simulink model "hpt_v2_1to1_switchlevel"  (R2025a)
settings: Solver=ode23tb  StartTime=0.0  StopTime=0.2  RelTol=1e-3
model workspace (MAT data in the model file):
  hpt_chopper_threshold = 850
  hpt_conventional_energy_scale = 1
  hpt_conventional_energy_scale_sag = 1
  hpt_conventional_energy_scale_swell = 1
  hpt_conventional_recovery_hold_s = 0
  hpt_conventional_recovery_reg_gain = 0
  hpt_conventional_recovery_reg_max = 0
  hpt_conventional_reg_scale = 1
  hpt_conventional_reg_scale_sag = 1
  hpt_conventional_reg_scale_swell = 1
  hpt_ctrl_Ts = 2e-05
  hpt_energy_bridge_polarity = -1
  hpt_energy_control_sign = -1
  hpt_energy_i_ki = 100
  hpt_energy_i_kp = 0.5
  hpt_energy_id_max = 20
  hpt_energy_openloop_amp = 0
  hpt_energy_openloop_phase = 0
  hpt_energy_vff_gain = 1.06
  hpt_grid_f0 = 50
  hpt_inj_phase_offset = -1.05
  hpt_m_energy = 0
  hpt_m_energy_max = 0.95
  hpt_m_reg = 0.1
  hpt_m_reg_max = 0.8
  hpt_pll_ki = 2500
  hpt_pll_kp = 80
  hpt_pwm_fs = 2000
  hpt_rchop = 5.33333333333
  hpt_sac_actor_filter_tau = 0.001
  hpt_sac_actor_select_mode = 0
  hpt_sac_dynamic_reg_limit = 0.8
  hpt_sac_enable = 0
  hpt_sac_energy_enable = 0
  hpt_sac_energy_max = 0.95
  hpt_sac_fault_time_norm_s = 0.5
  hpt_sac_fixed_energy_d = 0
  hpt_sac_fixed_energy_q = 0
  hpt_sac_fixed_reg_d = 0
  hpt_sac_fixed_reg_q = 0
  hpt_sac_grid_vref_phase = 5773.5026919
  hpt_sac_gridnorm_startup_s = 0.03
  hpt_sac_guard_enable = 0
  hpt_sac_i_base_peak = 816.496580928
  hpt_sac_phase_fault_clear_s = 0
  hpt_sac_phase_fault_start_s = 0
  hpt_sac_phase_override_enable = 0
  hpt_sac_phase_recovery_end_s = 0
  hpt_sac_policy_mode = 0
  hpt_sac_recovery_time_norm_s = 0.5
  hpt_sac_reg_d_gain = 1
  hpt_sac_reg_max = 0.8
  hpt_sac_reg_polarity = 1
  hpt_sac_reg_q_gain = 1
  hpt_sac_topology_id = 1
  hpt_sac_vdc_ref = 800
  hpt_sac_vref_phase = 230
  hpt_swell_gain_scale = 1
  hpt_traj_action = [0  0  0  0; 0  0  0  0; 0  0  0  0; 0  0  0  0; 0  0  0  0; 0  0  0  0; 0  0  0  0; 0  0  0  0; 0  0  0  0; 0  0  0  0; 0  0  0  0; 0  0  0  0; 0  0  0  0; 0  0  0  0; 0  0  0  0; 0  0  0  0; 0  0  0  0; 0  0  0  0; 0  0  0  0; 0  0  0  0; 0  0  0  0; 0  0  0  0; 0  0  0  0; 0  0  0  0; 0  0  0  0; 0  0  0  0; 0  0  0  0; 0  0  0  0; 0  0  0  0; 0  0  0  0; 0  0  0  0; 0  0  0  0; 0  0  0  0; 0  0  0  0; 0  0  0  0; 0  0  0  0; 0  0  0  0; 0  0  0  0; 0  0  0  0; 0  0  0  0; 0  0  0  0; 0  0  0  0; 0  0  0  0; 0  0  0  0; 0  0  0  0; 0  0  0  0; 0  0  0  0; 0  0  0  0; 0  0  0  0; 0  0  0  0; 0  0  0  0; 0  0  0  0; 0  0  0  0; 0  0  0  0; 0  0  0  0; 0  0  0  0; 0  0  0  0; 0  0  0  0; 0  0  0  0; 0  0  0  0; 0  0  0  0; 0  0  0  0; 0  0  0  0; 0  0  0  0; 0  0  0  0; 0  0  0  0; 0  0  0  0; 0  0  0  0; 0  0  0  0; 0  0  0  0; 0  0  0  0; 0  0  0  0; 0  0  0  0; 0  0  0  0; 0  0  0  0; 0  0  0  0; 0  0  0  0; 0  0  0  0; 0  0  0  0; 0  0  0  0; 0  0  0  0; 0  0  0  0; 0  0  0  0; 0  0  0  0; 0  0  0  0; 0  0  0  0; 0  0  0  0; 0  0  0  0; 0  0  0  0; 0  0  0  0; 0  0  0  0; 0  0  0  0; 0  0  0  0; 0  0  0  0; 0  0  0  0; 0  0  0  0; 0  0  0  0; 0  0  0  0; 0  0  0  0; 0  0  0  0; 0  0  0  0; 0  0  0  0; 0  0  0  0; 0  0  0  0; 0  0  0  0; 0  0  0  0; 0  0  0  0; 0  0  0  0; 0  0  0  0; 0  0  0  0; 0  0  0  0; 0  0  0  0; 0  0  0  0; 0  0  0  0; 0  0  0  0; 0  0  0  0; 0  0  0  0; 0  0  0  0; 0  0  0  0; 0  0  0  0; 0  0  0  0; 0  0  0  0; 0  0  0  0; 0  0  0  0; 0  0  0  0; 0  0  0  0]
  hpt_traj_t = [0; 0.002; 0.004; 0.006; 0.008; 0.01; 0.012; 0.014; 0.016; 0.018; 0.02; 0.022; 0.024; 0.026; 0.028; 0.03; 0.032; 0.034; 0.036; 0.038; 0.04; 0.042; 0.044; 0.046; 0.048; 0.05; 0.052; 0.054; 0.056; 0.058; 0.06; 0.062; 0.064; 0.066; 0.068; 0.07; 0.072; 0.074; 0.076; 0.078; 0.08; 0.082; 0.084; 0.086; 0.088; 0.09; 0.092; 0.094; 0.096; 0.098; 0.1; 0.102; 0.104; 0.106; 0.108; 0.11; 0.112; 0.114; 0.116; 0.118; 0.12; 0.122; 0.124; 0.126; 0.128; 0.13; 0.132; 0.134; 0.136; 0.138; 0.14; 0.142; 0.144; 0.146; 0.148; 0.15; 0.152; 0.154; 0.156; 0.158; 0.16; 0.162; 0.164; 0.166; 0.168; 0.17; 0.172; 0.174; 0.176; 0.178; 0.18; 0.182; 0.184; 0.186; 0.188; 0.19; 0.192; 0.194; 0.196; 0.198; 0.2; 0.202; 0.204; 0.206; 0.208; 0.21; 0.212; 0.214; 0.216; 0.218; 0.22; 0.222; 0.224; 0.226; 0.228; 0.23; 0.232; 0.234; 0.236; 0.238; 0.24; 0.242; 0.244; 0.246; 0.248; 0.25]
  hpt_vdc_ki = 0.2
  hpt_vdc_kp = 0.1
  hpt_vdc_ref = 800
  hpt_vref_lv = 207
  hpt_vreg_ki = 0
  hpt_vreg_kp = 20
libraries: simulink x9, spsLinearTransformerLib x9, spsUniversalBridgeLib x4, spsGroundLib x4, spsThreePhaseVIMeasurementLib x3, spsSeriesRLCBranchLib x2, spsThreePhaseSeriesRLCBranchLib x2, spsIGBTLib x1, spsVoltageMeasurementLib x1, spsThreePhaseSourceLib x1, spsThreePhaseSeriesRLCLoadLib x1, spspowerguiLib x1
(part 1 of 2)
settings Model: Creator=m1391  LastModifiedBy=m1391

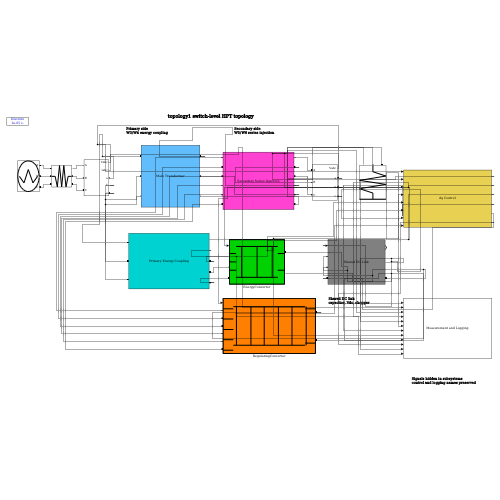
[thumbnail: Simulink's stored preview of the top-level diagram]
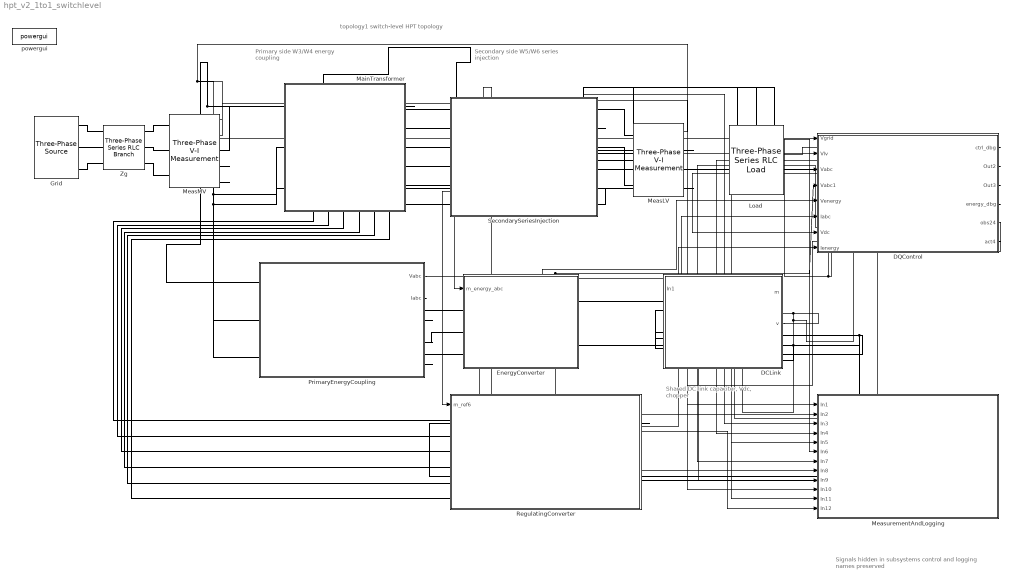
== system hpt_v2_1to1_switchlevel ==
  note: topology1 switch-level HPT topology
  note: Primary side
      | W3/W4 energy coupling
  note: Secondary side
      | W5/W6 series injection
  note: Shared DC link
      | capacitor, Vdc, chopper
  note: Signals hidden in subsystems
      | control and logging names preserved
  DCLink : Subsystem
      mask Display: disp('Shared DC Link');
  DQControl : Subsystem
      mask Display: disp('dq Control');
  EnergyConverter : Subsystem
      mask Display:
      | color('black');
      | plot([10 90 90 10 10],[10 10 90 90 10]);
      | plot([20 80],[78 78]); plot([20 80],[22 22]);
      | plot([28 28],[22 78]); plot([50 50],[22 78]); plot([72 72],[22 78]);
      | plot([10 20],[65 65]); plot([10 20],[50 50]); plot([10 20],[35 35]);
      | plot([80 90],[65 65]); plot([80 90],[35 35]);
  Grid : spsThreePhaseSourceLib/Three-Phase Source  InternalConnection=Yg  VoltagePhases=off  Voltage=10000  PhaseAngle=0  Voltage_phases=[25e3 25e3 25e3]/sqrt(3)  PhaseAngles_phases=[0 -120 +120]  Frequency=50  NonIdealSource=on  SpecifyImpedance=off  Resistance=1e-3  Inductance=1e-5  ShortCircuitLevel=100e6  BaseVoltage=25e3  XRratio=7  BusType=swing  Pref=10e3  Qref=0  Prefabc=[10e3, 10e3, 10e3]  Qrefabc=[0, 0, 0]  Qmin=-inf  Qmax=inf
  Load : spsThreePhaseSeriesRLCLoadLib/Three-Phase Series RLC Load  LConnTagsString=A|B|C  Configuration=Y (grounded)  NominalVoltage=400  Vabc=[1e3 1e3 1e3]  Vabcp=[1e3 1e3 1e3]  NominalFrequency=50  UnbalancedPower=off  ActivePower=400000  InductivePower=0  CapacitivePower=0  Pabc=[10e3 9e3 11e3]  QLabc=[100 90 110]  QCabc=[100 90 110]  Pabcp=[10e3 9e3 11e3]  QLabcp=[100 90 110]  QCabcp=[100 90 110]  Measurements=None  LoadType=constant Z
  MainTransformer : Subsystem
      mask Display: disp('Main Transformer');
  MeasLV : spsThreePhaseVIMeasurementLib/Three-Phase V-I Measurement  VoltageMeasurement=phase-to-ground  SetLabelV=off  LabelV=Vabc  Vpu=off  VpuLL=off  CurrentMeasurement=no  SetLabelI=off  LabelI=Iabc  Ipu=off  Pbase=100e6  Vbase=500e3  OutputType=Complex  PhasorSimulation=off  PSBequivalent=0
  MeasMV : spsThreePhaseVIMeasurementLib/Three-Phase V-I Measurement  VoltageMeasurement=phase-to-ground  SetLabelV=off  LabelV=Vabc  Vpu=off  VpuLL=off  CurrentMeasurement=yes  SetLabelI=off  LabelI=Iabc  Ipu=off  Pbase=100e6  Vbase=500e3  OutputType=Complex  PhasorSimulation=off  PSBequivalent=0
  MeasurementAndLogging : Subsystem
      mask Display: disp('Measurement and Logging');
  PrimaryEnergyCoupling : Subsystem
      mask Display: disp('Primary Energy Coupling');
  RegulatingConverter : Subsystem
      mask Display:
      | color('black');
      | plot([5 95 95 5 5],[10 10 90 90 10]);
      | plot([15 85],[78 78]); plot([15 85],[22 22]);
      | plot([18 18],[22 78]); plot([32 32],[22 78]);
      | plot([45 45],[22 78]); plot([59 59],[22 78]);
      | plot([72 72],[22 78]); plot([86 86],[22 78]);
      | plot([5 15],[75 75]); plot([5 15],[60 60]); plot([5 15],[45 45]);
      | plot([5 15],[30 30]); plot([5 15],[15 15]); plot([5 15],[10 10]);
      | plot([85 95],[75 75]); plot([85 95],[25 25]);
  SecondarySeriesInjection : Subsystem
      mask Display: disp('Secondary Series Injection');
  Zg : spsThreePhaseSeriesRLCBranchLib/Three-Phase Series RLC Branch  LConnTagsString=A|B|C  RConnTagsString=A|B|C  BranchType=RL  Resistance=11.7851  Inductance=0.26259  Capacitance=1e-6  Measurements=None
  powergui : spspowerguiLib/powergui  Priority=1  SimulationMode=Discrete  SampleTime=2e-05  frequency=60  Iterations=50  frequencyindice=60  Pbase=100e6  ErrMax=1e-4  UnitsV=kV  UnitsW=MW  buscounter=0  FunctionMessages=off  echomessages=off  EnableUseOfTLC=off  CurrentSourceSwitches=off  DisableSnubberDevices=off  DisableRonSwitches=off  DisableVfSwitches=off  DisplayEquations=off  AutomaticDiscreteSolvers=off  SolverType=Tustin/Backward Euler (TBE)  Interpol=off  ExternalGateDelay=off  methode=off  Ts=100  x0status=blocks  SPID=on  SwTol=0  HookPort=off  NonlinearTolerance=1e-4  nMaxIteration=100  ContinueOnMaxIteration=off  RestoreLinks=warning  ResistiveCurrentMeasurement=off  Frange=[0:2:500]  Ylog=off  Xlog=on  ShowGrid=off  save=off  variable=ZData  structure=0  ZoomFFT=off  StartTime=0.0  cycles=1  DisplayStyle=1  fundamental=60  FreqAxis=off  MaxFrequency=1000  frequencyindicesteady=1  RmsSteady=1  display=off
  wires:
  MeasMV/1 -> MeasurementAndLogging/1(In1), DQControl/1(Vgrid)
  MeasLV/1 -> DQControl/2(Vlv), MeasurementAndLogging/3(In3), DQControl/3(Vabc)
  PrimaryEnergyCoupling/1(Vabc) -> DQControl/5(Venergy), MeasurementAndLogging/8(In8), DQControl/4(Vabc1)
  PrimaryEnergyCoupling/2(Iabc) -> DQControl/6(Iabc), MeasurementAndLogging/12(In12), DQControl/8(Ienergy)
  DQControl/3(Out3) -> MeasurementAndLogging/6(In6), EnergyConverter/1(m_energy_abc)
  DQControl/2(Out2) -> MeasurementAndLogging/4(In4), RegulatingConverter/1(m_ref6)
  DCLink/2(v) -> MeasurementAndLogging/11(In11), DCLink/1(In1), DQControl/7(Vdc)
  MeasMV/2 -> MeasurementAndLogging/2(In2)
  DQControl/1(ctrl_dbg) -> MeasurementAndLogging/5(In5)
  DQControl/4(energy_dbg) -> MeasurementAndLogging/7(In7)
  DQControl/5(obs24) -> MeasurementAndLogging/9(In9)
  DQControl/6(act4) -> MeasurementAndLogging/10(In10)
  connections:
  Grid/RConn1 -- Zg/LConn1
  Zg/RConn1 -- MeasMV/LConn1
  MeasMV/RConn1 -- PrimaryEnergyCoupling/LConn1 -- MainTransformer/LConn1
  MeasLV/RConn1 -- Load/LConn1
  Grid/RConn2 -- Zg/LConn2
  Zg/RConn2 -- MeasMV/LConn2
  MeasMV/RConn2 -- PrimaryEnergyCoupling/LConn2 -- MainTransformer/LConn2
  MeasLV/RConn2 -- Load/LConn2
  Grid/RConn3 -- Zg/LConn3
  Zg/RConn3 -- MeasMV/LConn3
  MeasLV/RConn3 -- Load/LConn3
  MeasMV/RConn3 -- PrimaryEnergyCoupling/LConn3 -- MainTransformer/LConn3
  PrimaryEnergyCoupling/RConn1 -- EnergyConverter/LConn1
  PrimaryEnergyCoupling/RConn2 -- EnergyConverter/LConn2
  PrimaryEnergyCoupling/RConn3 -- EnergyConverter/LConn3
  SecondarySeriesInjection/RConn1 -- MeasLV/LConn1
  SecondarySeriesInjection/RConn2 -- MeasLV/LConn2
  SecondarySeriesInjection/RConn3 -- MeasLV/LConn3
  MainTransformer/RConn1 -- SecondarySeriesInjection/RConn4
  MainTransformer/RConn2 -- SecondarySeriesInjection/RConn5
  MainTransformer/RConn3 -- SecondarySeriesInjection/RConn6
  SecondarySeriesInjection/LConn1 -- RegulatingConverter/LConn1
  SecondarySeriesInjection/LConn2 -- RegulatingConverter/LConn2
  SecondarySeriesInjection/LConn3 -- RegulatingConverter/LConn3
  SecondarySeriesInjection/LConn4 -- RegulatingConverter/LConn4
  SecondarySeriesInjection/LConn5 -- RegulatingConverter/LConn5
  SecondarySeriesInjection/LConn6 -- RegulatingConverter/LConn6
  RegulatingConverter/RConn1 -- DCLink/LConn3 -- EnergyConverter/RConn1 -- DCLink/LConn1
  EnergyConverter/RConn2 -- DCLink/RConn1 -- RegulatingConverter/RConn2 -- DCLink/LConn2

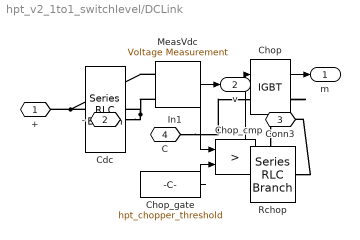
== system hpt_v2_1to1_switchlevel/DCLink ==
  In1 : Inport
  Cdc : spsSeriesRLCBranchLib/Series RLC Branch  LConnTagsString=__new0  RConnTagsString=__new0  BranchType=C  Resistance=1  Inductance=1e-3  SetiL0=off  InitialCurrent=0  Capacitance=0.0022  Setx0=on  InitialVoltage=800  Measurements=None
  Chop : spsIGBTLib/IGBT  Ron=0.001  Lon=0  Vf=1  Tf=1e-6  Tt=2e-6  IC=0  Rs=1e5  Cs=inf  Measurements=on
  Chop_cmp : RelationalOperator  Operator=>  OutDataTypeStr=boolean  RndMeth=Simplest  InputSameDT=off
  Chop_gate : Constant  Value=hpt_chopper_threshold
      mask Display: plot([20 80 80 20 20],[30 30 70 70 30]);
  MeasVdc : spsVoltageMeasurementLib/Voltage Measurement  PhasorSimulation=off  OutputType=Complex  PSBequivalent=0
  Rchop : spsSeriesRLCBranchLib/Series RLC Branch  LConnTagsString=__new0  RConnTagsString=__new0  BranchType=R  Resistance=hpt_rchop  Inductance=1e-3  SetiL0=off  InitialCurrent=0  Capacitance=1e-6  Setx0=off  InitialVoltage=0  Measurements=None
  + : PMIOPort  Side=Left
  - : PMIOPort  Port=2  Side=Left
  Conn3 : PMIOPort  Port=3  Side=Right
  C : PMIOPort  Port=4  Side=Left
  m : Outport
  v : Outport  Port=2
  wires:
  In1/1 -> Chop_cmp/1
  Chop_cmp/1 -> Chop/1
  Chop_gate/1 -> Chop_cmp/2
  MeasVdc/1 -> v/1
  Chop/1 -> m/1
  connections:
  MeasVdc/LConn2 -- -/RConn1 -- Cdc/RConn1
  C/RConn1 -- Chop/LConn1
  Cdc/LConn1 -- +/RConn1 -- MeasVdc/LConn1
  Chop/RConn1 -- Rchop/LConn1
  Rchop/RConn1 -- Conn3/RConn1

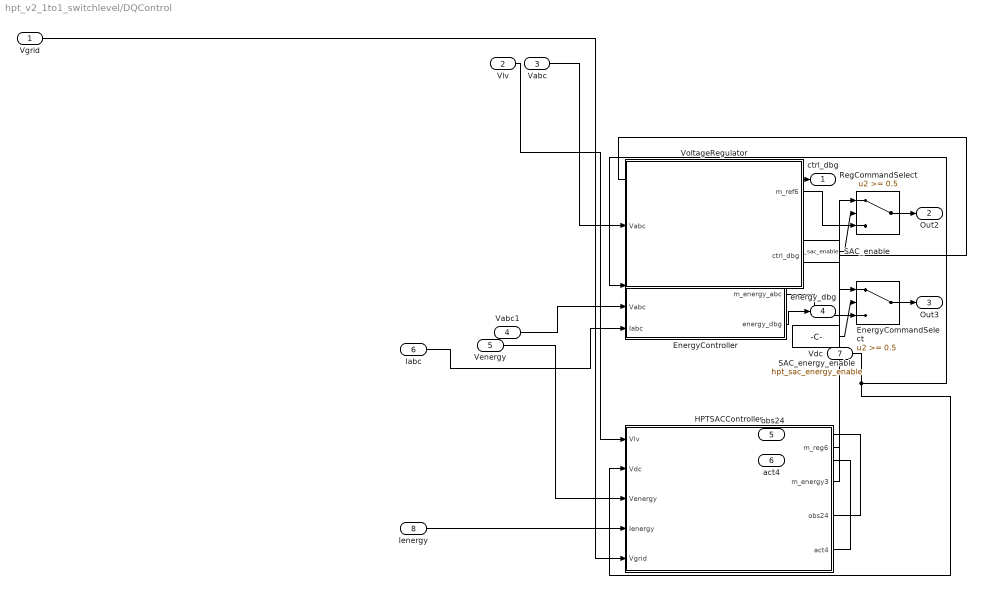
== system hpt_v2_1to1_switchlevel/DQControl ==
  Vgrid : Inport
  Vlv : Inport  Port=2
  Vabc : Inport  Port=3
  Vabc1 : Inport  Port=4
  Venergy : Inport  Port=5
  Iabc : Inport  Port=6
  Vdc : Inport  Port=7
  Ienergy : Inport  Port=8
  EnergyCommandSelect : Switch  Threshold=0.5  SaturateOnIntegerOverflow=off  InputSameDT=off
  EnergyController : Subsystem
  HPTSACController : Subsystem
  RegCommandSelect : Switch  Threshold=0.5  SaturateOnIntegerOverflow=off  InputSameDT=off
  SAC_enable : Constant  Value=hpt_sac_enable
      mask Display: plot([20 80 80 20 20],[30 30 70 70 30]);
  SAC_energy_enable : Constant  Value=hpt_sac_energy_enable
      mask Display: plot([20 80 80 20 20],[30 30 70 70 30]);
  VoltageRegulator : Subsystem
  ctrl_dbg : Outport
  Out2 : Outport  Port=2
  Out3 : Outport  Port=3
  energy_dbg : Outport  Port=4
  obs24 : Outport  Port=5
  act4 : Outport  Port=6
  wires:
  VoltageRegulator/1(m_ref6) -> RegCommandSelect/3
  SAC_enable/1 -> RegCommandSelect/2
  Vdc/1 -> HPTSACController/2(Vdc), EnergyController/1(Vdc)
  HPTSACController/1(m_reg6) -> RegCommandSelect/1
  SAC_energy_enable/1 -> EnergyCommandSelect/2
  HPTSACController/2(m_energy3) -> EnergyCommandSelect/1
  EnergyController/1(m_energy_abc) -> EnergyCommandSelect/3
  EnergyController/2(energy_dbg) -> energy_dbg/1
  VoltageRegulator/2(ctrl_dbg) -> ctrl_dbg/1
  RegCommandSelect/1 -> Out2/1
  Vlv/1 -> HPTSACController/1(Vlv)
  HPTSACController/3(obs24) -> obs24/1
  EnergyCommandSelect/1 -> Out3/1
  Vabc/1 -> VoltageRegulator/1(Vabc)
  Vgrid/1 -> HPTSACController/5(Vgrid)
  Venergy/1 -> HPTSACController/3(Venergy)
  Ienergy/1 -> HPTSACController/4(Ienergy)
  Iabc/1 -> EnergyController/3(Iabc)
  HPTSACController/4(act4) -> act4/1
  Vabc1/1 -> EnergyController/2(Vabc)

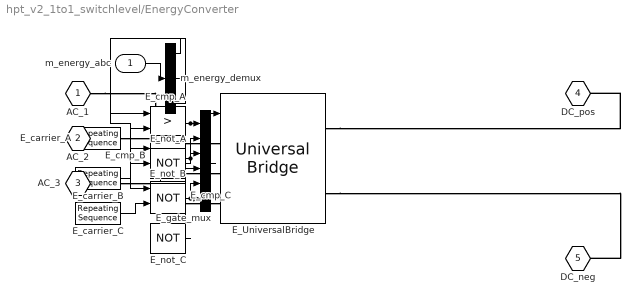
== system hpt_v2_1to1_switchlevel/EnergyConverter ==
  m_energy_abc : Inport
  E_UniversalBridge : spsUniversalBridgeLib/Universal Bridge  Arms=3  SnubberResistance=1e5  SnubberCapacitance=inf  Device=IGBT / Diodes  Ron=1e-3  Lon=0  ForwardVoltages=[0.8 0.8]  ForwardVoltage=0  GTOparameters=[ 10e-6 , 20e-6 ]  IGBTparameters=[ 1e-6 , 2e-6 ]  Measurements=None  Measurements_2=None  converterType=Rectifier
  E_carrier_A : simulink/Sources/Repeating Sequence  rep_seq_t=[0 0.5/hpt_pwm_fs 1/hpt_pwm_fs]  rep_seq_y=[-1 1 -1]
  E_carrier_B : simulink/Sources/Repeating Sequence  rep_seq_t=[0 0.5/hpt_pwm_fs 1/hpt_pwm_fs]  rep_seq_y=[-1 1 -1]
  E_carrier_C : simulink/Sources/Repeating Sequence  rep_seq_t=[0 0.5/hpt_pwm_fs 1/hpt_pwm_fs]  rep_seq_y=[-1 1 -1]
  E_cmp_A : RelationalOperator  Operator=>  OutDataTypeStr=boolean  RndMeth=Simplest  InputSameDT=off
  E_cmp_B : RelationalOperator  Operator=>  OutDataTypeStr=boolean  RndMeth=Simplest  InputSameDT=off
  E_cmp_C : RelationalOperator  Operator=>  OutDataTypeStr=boolean  RndMeth=Simplest  InputSameDT=off
  E_gate_mux : Mux  Inputs=6
  E_not_A : Logic  Operator=NOT  AllPortsSameDT=off  OutDataTypeStr=boolean
  E_not_B : Logic  Operator=NOT  AllPortsSameDT=off  OutDataTypeStr=boolean
  E_not_C : Logic  Operator=NOT  AllPortsSameDT=off  OutDataTypeStr=boolean
  m_energy_demux : Demux  Outputs=3
  AC_1 : PMIOPort  Side=Left
  AC_2 : PMIOPort  Port=2  Side=Left
  AC_3 : PMIOPort  Port=3  Side=Left
  DC_pos : PMIOPort  Port=4  Side=Right
  DC_neg : PMIOPort  Port=5  Side=Right
  wires:
  m_energy_abc/1 -> m_energy_demux/1
  m_energy_demux/1 -> E_cmp_A/1
  E_carrier_A/1 -> E_cmp_A/2
  E_cmp_A/1 -> E_gate_mux/1, E_not_A/1
  E_not_A/1 -> E_gate_mux/2
  m_energy_demux/2 -> E_cmp_B/1
  E_carrier_B/1 -> E_cmp_B/2
  E_cmp_B/1 -> E_gate_mux/3, E_not_B/1
  E_not_B/1 -> E_gate_mux/4
  m_energy_demux/3 -> E_cmp_C/1
  E_carrier_C/1 -> E_cmp_C/2
  E_cmp_C/1 -> E_gate_mux/5, E_not_C/1
  E_not_C/1 -> E_gate_mux/6
  E_gate_mux/1 -> E_UniversalBridge/1
  connections:
  AC_1/RConn1 -- E_UniversalBridge/LConn1
  AC_2/RConn1 -- E_UniversalBridge/LConn2
  AC_3/RConn1 -- E_UniversalBridge/LConn3
  E_UniversalBridge/RConn1 -- DC_pos/RConn1
  E_UniversalBridge/RConn2 -- DC_neg/RConn1

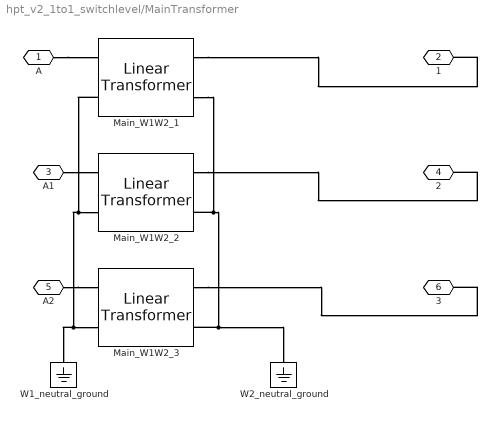
== system hpt_v2_1to1_switchlevel/MainTransformer ==
  Main_W1W2_1 : spsLinearTransformerLib/Linear Transformer  UNITS=pu  NominalPower=[133333.3333,50]  winding1=[5773.5027,0.005,0.025]  winding2=[230.9401,0.005,0.025]  ThreeWindings=off  winding3=[ 315e3 0.002 0.08 ]  RmLm=[ 500 500 ]  Measurements=None  DataType=off
  Main_W1W2_2 : spsLinearTransformerLib/Linear Transformer  UNITS=pu  NominalPower=[133333.3333,50]  winding1=[5773.5027,0.005,0.025]  winding2=[230.9401,0.005,0.025]  ThreeWindings=off  winding3=[ 315e3 0.002 0.08 ]  RmLm=[ 500 500 ]  Measurements=None  DataType=off
  Main_W1W2_3 : spsLinearTransformerLib/Linear Transformer  UNITS=pu  NominalPower=[133333.3333,50]  winding1=[5773.5027,0.005,0.025]  winding2=[230.9401,0.005,0.025]  ThreeWindings=off  winding3=[ 315e3 0.002 0.08 ]  RmLm=[ 500 500 ]  Measurements=None  DataType=off
  W1_neutral_ground : spsGroundLib/Ground  LConnTagsString=a
  W2_neutral_ground : spsGroundLib/Ground  LConnTagsString=a
  A : PMIOPort  Side=Left
  1 : PMIOPort  Port=2  Side=Right
  A1 : PMIOPort  Port=3  Side=Left
  2 : PMIOPort  Port=4  Side=Right
  A2 : PMIOPort  Port=5  Side=Left
  3 : PMIOPort  Port=6  Side=Right
  connections:
  Main_W1W2_2/RConn1 -- 2/RConn1
  Main_W1W2_1/LConn2 -- Main_W1W2_2/LConn2 -- Main_W1W2_3/LConn2 -- W1_neutral_ground/LConn1
  A/RConn1 -- Main_W1W2_1/LConn1
  A1/RConn1 -- Main_W1W2_2/LConn1
  Main_W1W2_1/RConn2 -- Main_W1W2_2/RConn2 -- Main_W1W2_3/RConn2 -- W2_neutral_ground/LConn1
  A2/RConn1 -- Main_W1W2_3/LConn1
  Main_W1W2_1/RConn1 -- 1/RConn1
  Main_W1W2_3/RConn1 -- 3/RConn1

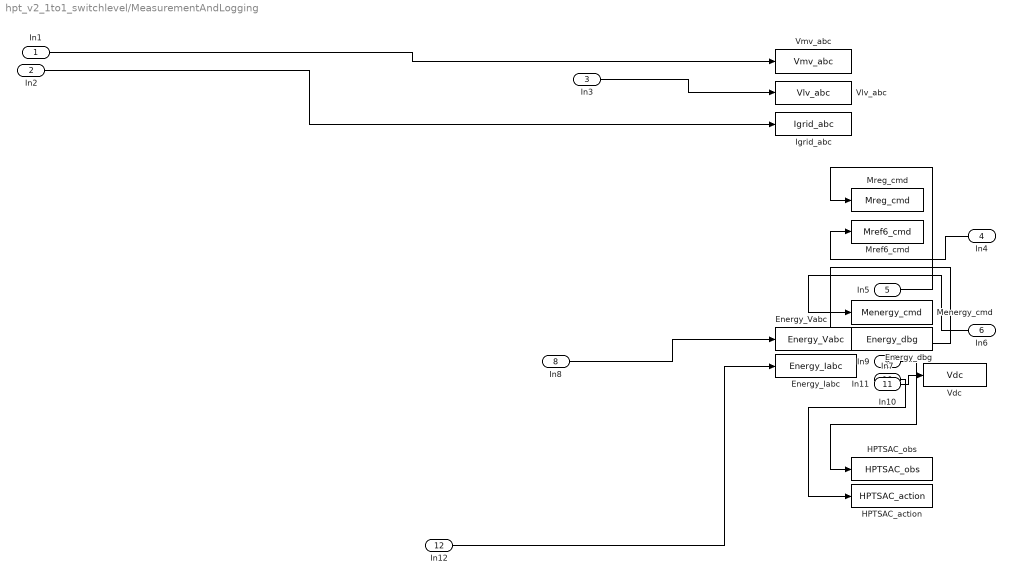
== system hpt_v2_1to1_switchlevel/MeasurementAndLogging ==
  In1 : Inport
  In2 : Inport  Port=2
  In3 : Inport  Port=3
  In4 : Inport  Port=4
  In5 : Inport  Port=5
  In6 : Inport  Port=6
  In7 : Inport  Port=7
  In8 : Inport  Port=8
  In9 : Inport  Port=9
  In10 : Inport  Port=10
  In11 : Inport  Port=11
  In12 : Inport  Port=12
  Energy_Iabc : ToWorkspace  VariableName=Energy_Iabc  SampleTime=2e-05
      mask Display: plot([10 90 90 10 10],[25 25 75 75 25]);
  Energy_Vabc : ToWorkspace  VariableName=Energy_Vabc  SampleTime=2e-05
      mask Display: plot([10 90 90 10 10],[25 25 75 75 25]);
  Energy_dbg : ToWorkspace  VariableName=Energy_dbg  SampleTime=2e-05
      mask Display: plot([10 90 90 10 10],[25 25 75 75 25]);
  HPTSAC_action : ToWorkspace  VariableName=HPTSAC_action  SampleTime=2e-05
      mask Display: plot([10 90 90 10 10],[25 25 75 75 25]);
  HPTSAC_obs : ToWorkspace  VariableName=HPTSAC_obs  SampleTime=2e-05
      mask Display: plot([10 90 90 10 10],[25 25 75 75 25]);
  Igrid_abc : ToWorkspace  VariableName=Igrid_abc  SampleTime=2e-05
      mask Display: plot([10 90 90 10 10],[25 25 75 75 25]);
  Menergy_cmd : ToWorkspace  VariableName=Menergy_cmd  SampleTime=2e-05
      mask Display: plot([10 90 90 10 10],[25 25 75 75 25]);
  Mref6_cmd : ToWorkspace  VariableName=Mref6_cmd  SampleTime=2e-05
      mask Display: plot([10 90 90 10 10],[25 25 75 75 25]);
  Mreg_cmd : ToWorkspace  VariableName=Mreg_cmd  SampleTime=2e-05
      mask Display: plot([10 90 90 10 10],[25 25 75 75 25]);
  Vdc : ToWorkspace  VariableName=Vdc  SampleTime=2e-05
      mask Display: plot([10 90 90 10 10],[25 25 75 75 25]);
  Vlv_abc : ToWorkspace  VariableName=Vlv_abc  SampleTime=2e-05
      mask Display: plot([10 90 90 10 10],[25 25 75 75 25]);
  Vmv_abc : ToWorkspace  VariableName=Vmv_abc  SampleTime=2e-05
      mask Display: plot([10 90 90 10 10],[25 25 75 75 25]);
  wires:
  In10/1 -> HPTSAC_action/1
  In11/1 -> Vdc/1
  In2/1 -> Igrid_abc/1
  In8/1 -> Energy_Vabc/1
  In4/1 -> Mref6_cmd/1
  In1/1 -> Vmv_abc/1
  In12/1 -> Energy_Iabc/1
  In9/1 -> HPTSAC_obs/1
  In3/1 -> Vlv_abc/1
  In5/1 -> Mreg_cmd/1
  In7/1 -> Energy_dbg/1
  In6/1 -> Menergy_cmd/1

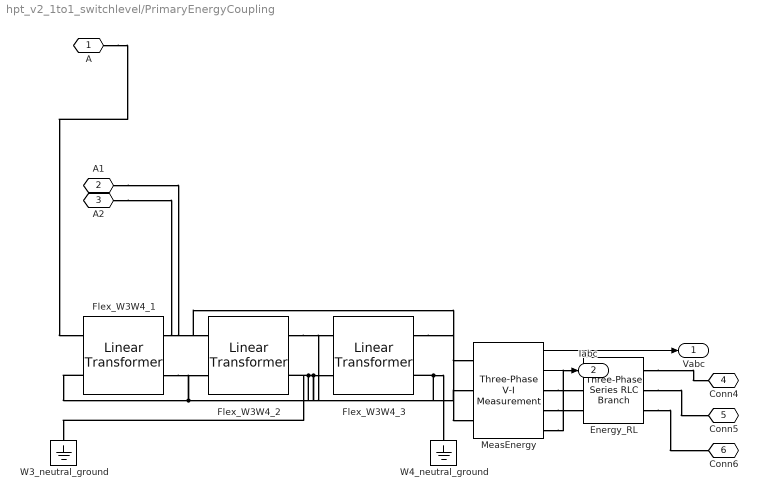
== system hpt_v2_1to1_switchlevel/PrimaryEnergyCoupling ==
  Energy_RL : spsThreePhaseSeriesRLCBranchLib/Three-Phase Series RLC Branch  LConnTagsString=A|B|C  RConnTagsString=A|B|C  BranchType=RL  Resistance=0.05  Inductance=0.003  Capacitance=1e-6  Measurements=None
  Flex_W3W4_1 : spsLinearTransformerLib/Linear Transformer  UNITS=pu  NominalPower=[40000,50]  winding1=[5773.5027,0.005,0.02]  winding2=[230.9401,0.005,0.02]  ThreeWindings=off  winding3=[ 315e3 0.002 0.08 ]  RmLm=[ 500 500 ]  Measurements=None  DataType=off
  Flex_W3W4_2 : spsLinearTransformerLib/Linear Transformer  UNITS=pu  NominalPower=[40000,50]  winding1=[5773.5027,0.005,0.02]  winding2=[230.9401,0.005,0.02]  ThreeWindings=off  winding3=[ 315e3 0.002 0.08 ]  RmLm=[ 500 500 ]  Measurements=None  DataType=off
  Flex_W3W4_3 : spsLinearTransformerLib/Linear Transformer  UNITS=pu  NominalPower=[40000,50]  winding1=[5773.5027,0.005,0.02]  winding2=[230.9401,0.005,0.02]  ThreeWindings=off  winding3=[ 315e3 0.002 0.08 ]  RmLm=[ 500 500 ]  Measurements=None  DataType=off
  MeasEnergy : spsThreePhaseVIMeasurementLib/Three-Phase V-I Measurement  VoltageMeasurement=phase-to-ground  SetLabelV=off  LabelV=Vabc  Vpu=off  VpuLL=off  CurrentMeasurement=yes  SetLabelI=off  LabelI=Iabc  Ipu=off  Pbase=100e6  Vbase=500e3  OutputType=Complex  PhasorSimulation=off  PSBequivalent=0
  W3_neutral_ground : spsGroundLib/Ground  LConnTagsString=a
  W4_neutral_ground : spsGroundLib/Ground  LConnTagsString=a
  A : PMIOPort  Side=Left
  A1 : PMIOPort  Port=2  Side=Left
  A2 : PMIOPort  Port=3  Side=Left
  Conn4 : PMIOPort  Port=4  Side=Right
  Conn5 : PMIOPort  Port=5  Side=Right
  Conn6 : PMIOPort  Port=6  Side=Right
  Vabc : Outport
  Iabc : Outport  Port=2
  wires:
  MeasEnergy/1 -> Vabc/1
  MeasEnergy/2 -> Iabc/1
  connections:
  Flex_W3W4_3/RConn1 -- MeasEnergy/LConn3
  Flex_W3W4_2/RConn1 -- MeasEnergy/LConn2
  A1/RConn1 -- Flex_W3W4_2/LConn1
  Flex_W3W4_1/RConn2 -- Flex_W3W4_2/RConn2 -- Flex_W3W4_3/RConn2 -- W4_neutral_ground/LConn1
  A2/RConn1 -- Flex_W3W4_3/LConn1
  Flex_W3W4_1/RConn1 -- MeasEnergy/LConn1
  Flex_W3W4_1/LConn2 -- Flex_W3W4_2/LConn2 -- Flex_W3W4_3/LConn2 -- W3_neutral_ground/LConn1
  Energy_RL/RConn2 -- Conn5/RConn1
  MeasEnergy/RConn3 -- Energy_RL/LConn3
  MeasEnergy/RConn1 -- Energy_RL/LConn1
  MeasEnergy/RConn2 -- Energy_RL/LConn2
  A/RConn1 -- Flex_W3W4_1/LConn1
  Energy_RL/RConn1 -- Conn4/RConn1
  Energy_RL/RConn3 -- Conn6/RConn1

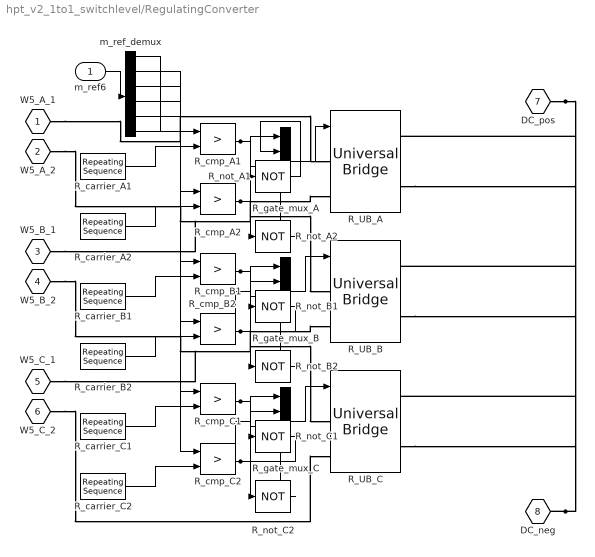
== system hpt_v2_1to1_switchlevel/RegulatingConverter ==
  m_ref6 : Inport
  R_UB_A : spsUniversalBridgeLib/Universal Bridge  Arms=2  SnubberResistance=1e5  SnubberCapacitance=1e-9  Device=IGBT / Diodes  Ron=1e-3  Lon=0  ForwardVoltages="[  0  0  ]"  ForwardVoltage=0  GTOparameters=[ 10e-6 , 20e-6 ]  IGBTparameters=[ 1e-6 , 2e-6 ]  Measurements=None  Measurements_2=None  converterType=Rectifier
  R_UB_B : spsUniversalBridgeLib/Universal Bridge  Arms=2  SnubberResistance=1e5  SnubberCapacitance=1e-9  Device=IGBT / Diodes  Ron=1e-3  Lon=0  ForwardVoltages="[  0  0  ]"  ForwardVoltage=0  GTOparameters=[ 10e-6 , 20e-6 ]  IGBTparameters=[ 1e-6 , 2e-6 ]  Measurements=None  Measurements_2=None  converterType=Rectifier
  R_UB_C : spsUniversalBridgeLib/Universal Bridge  Arms=2  SnubberResistance=1e5  SnubberCapacitance=1e-9  Device=IGBT / Diodes  Ron=1e-3  Lon=0  ForwardVoltages="[  0  0  ]"  ForwardVoltage=0  GTOparameters=[ 10e-6 , 20e-6 ]  IGBTparameters=[ 1e-6 , 2e-6 ]  Measurements=None  Measurements_2=None  converterType=Rectifier
  R_carrier_A1 : simulink/Sources/Repeating Sequence  rep_seq_t=[0 0.5/hpt_pwm_fs 1/hpt_pwm_fs]  rep_seq_y=[-1 1 -1]
  R_carrier_A2 : simulink/Sources/Repeating Sequence  rep_seq_t=[0 0.5/hpt_pwm_fs 1/hpt_pwm_fs]  rep_seq_y=[-1 1 -1]
  R_carrier_B1 : simulink/Sources/Repeating Sequence  rep_seq_t=[0 0.5/hpt_pwm_fs 1/hpt_pwm_fs]  rep_seq_y=[-1 1 -1]
  R_carrier_B2 : simulink/Sources/Repeating Sequence  rep_seq_t=[0 0.5/hpt_pwm_fs 1/hpt_pwm_fs]  rep_seq_y=[-1 1 -1]
  R_carrier_C1 : simulink/Sources/Repeating Sequence  rep_seq_t=[0 0.5/hpt_pwm_fs 1/hpt_pwm_fs]  rep_seq_y=[-1 1 -1]
  R_carrier_C2 : simulink/Sources/Repeating Sequence  rep_seq_t=[0 0.5/hpt_pwm_fs 1/hpt_pwm_fs]  rep_seq_y=[-1 1 -1]
  R_cmp_A1 : RelationalOperator  Operator=>  OutDataTypeStr=boolean  RndMeth=Simplest  InputSameDT=off
  R_cmp_A2 : RelationalOperator  Operator=>  OutDataTypeStr=boolean  RndMeth=Simplest  InputSameDT=off
  R_cmp_B1 : RelationalOperator  Operator=>  OutDataTypeStr=boolean  RndMeth=Simplest  InputSameDT=off
  R_cmp_B2 : RelationalOperator  Operator=>  OutDataTypeStr=boolean  RndMeth=Simplest  InputSameDT=off
  R_cmp_C1 : RelationalOperator  Operator=>  OutDataTypeStr=boolean  RndMeth=Simplest  InputSameDT=off
  R_cmp_C2 : RelationalOperator  Operator=>  OutDataTypeStr=boolean  RndMeth=Simplest  InputSameDT=off
  R_gate_mux_A : Mux
  R_gate_mux_B : Mux
  R_gate_mux_C : Mux
  R_not_A1 : Logic  Operator=NOT  AllPortsSameDT=off  OutDataTypeStr=boolean
  R_not_A2 : Logic  Operator=NOT  AllPortsSameDT=off  OutDataTypeStr=boolean
  R_not_B1 : Logic  Operator=NOT  AllPortsSameDT=off  OutDataTypeStr=boolean
  R_not_B2 : Logic  Operator=NOT  AllPortsSameDT=off  OutDataTypeStr=boolean
  R_not_C1 : Logic  Operator=NOT  AllPortsSameDT=off  OutDataTypeStr=boolean
  R_not_C2 : Logic  Operator=NOT  AllPortsSameDT=off  OutDataTypeStr=boolean
  m_ref_demux : Demux  Outputs=6
  W5_A_1 : PMIOPort  Side=Left
  W5_A_2 : PMIOPort  Port=2  Side=Left
  W5_B_1 : PMIOPort  Port=3  Side=Left
  W5_B_2 : PMIOPort  Port=4  Side=Left
  W5_C_1 : PMIOPort  Port=5  Side=Left
  W5_C_2 : PMIOPort  Port=6  Side=Left
  DC_pos : PMIOPort  Port=7  Side=Right
  DC_neg : PMIOPort  Port=8  Side=Right
  wires:
  m_ref6/1 -> m_ref_demux/1
  m_ref_demux/1 -> R_cmp_A1/1
  R_carrier_A1/1 -> R_cmp_A1/2
  R_cmp_A1/1 -> R_gate_mux_A/1, R_not_A1/1
  R_not_A1/1 -> R_gate_mux_A/2
  m_ref_demux/2 -> R_cmp_A2/1
  R_carrier_A2/1 -> R_cmp_A2/2
  R_cmp_A2/1 -> R_gate_mux_A/3, R_not_A2/1
  R_not_A2/1 -> R_gate_mux_A/4
  R_gate_mux_A/1 -> R_UB_A/1
  m_ref_demux/3 -> R_cmp_B1/1
  R_carrier_B1/1 -> R_cmp_B1/2
  R_cmp_B1/1 -> R_gate_mux_B/1, R_not_B1/1
  R_not_B1/1 -> R_gate_mux_B/2
  m_ref_demux/4 -> R_cmp_B2/1
  R_carrier_B2/1 -> R_cmp_B2/2
  R_cmp_B2/1 -> R_gate_mux_B/3, R_not_B2/1
  R_not_B2/1 -> R_gate_mux_B/4
  R_gate_mux_B/1 -> R_UB_B/1
  m_ref_demux/5 -> R_cmp_C1/1
  R_carrier_C1/1 -> R_cmp_C1/2
  R_cmp_C1/1 -> R_gate_mux_C/1, R_not_C1/1
  R_not_C1/1 -> R_gate_mux_C/2
  m_ref_demux/6 -> R_cmp_C2/1
  R_carrier_C2/1 -> R_cmp_C2/2
  R_cmp_C2/1 -> R_gate_mux_C/3, R_not_C2/1
  R_not_C2/1 -> R_gate_mux_C/4
  R_gate_mux_C/1 -> R_UB_C/1
  connections:
  W5_A_1/RConn1 -- R_UB_A/LConn1
  W5_A_2/RConn1 -- R_UB_A/LConn2
  W5_B_1/RConn1 -- R_UB_B/LConn1
  W5_B_2/RConn1 -- R_UB_B/LConn2
  W5_C_1/RConn1 -- R_UB_C/LConn1
  W5_C_2/RConn1 -- R_UB_C/LConn2
  R_UB_A/RConn1 -- DC_pos/RConn1 -- R_UB_B/RConn1 -- R_UB_C/RConn1
  R_UB_A/RConn2 -- R_UB_B/RConn2 -- DC_neg/RConn1 -- R_UB_C/RConn2

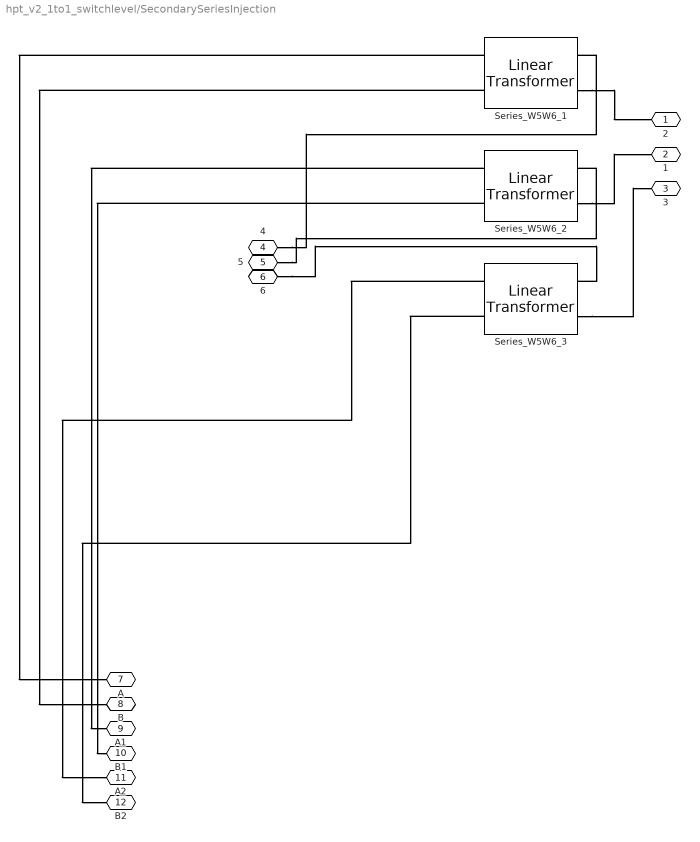
== system hpt_v2_1to1_switchlevel/SecondarySeriesInjection ==
  Series_W5W6_1 : spsLinearTransformerLib/Linear Transformer  UNITS=pu  NominalPower=[30000,50]  winding1=[400,0.002,0.03]  winding2=[100,0.002,0.03]  ThreeWindings=off  winding3=[ 315e3 0.002 0.08 ]  RmLm=[ 500 500 ]  Measurements=None  DataType=off
  Series_W5W6_2 : spsLinearTransformerLib/Linear Transformer  UNITS=pu  NominalPower=[30000,50]  winding1=[400,0.002,0.03]  winding2=[100,0.002,0.03]  ThreeWindings=off  winding3=[ 315e3 0.002 0.08 ]  RmLm=[ 500 500 ]  Measurements=None  DataType=off
  Series_W5W6_3 : spsLinearTransformerLib/Linear Transformer  UNITS=pu  NominalPower=[30000,50]  winding1=[400,0.002,0.03]  winding2=[100,0.002,0.03]  ThreeWindings=off  winding3=[ 315e3 0.002 0.08 ]  RmLm=[ 500 500 ]  Measurements=None  DataType=off
  2 : PMIOPort  Side=Right
  1 : PMIOPort  Port=2  Side=Right
  3 : PMIOPort  Port=3  Side=Right
  4 : PMIOPort  Port=4  Side=Right
  5 : PMIOPort  Port=5  Side=Right
  6 : PMIOPort  Port=6  Side=Right
  A : PMIOPort  Port=7  Side=Left
  B : PMIOPort  Port=8  Side=Left
  A1 : PMIOPort  Port=9  Side=Left
  B1 : PMIOPort  Port=10  Side=Left
  A2 : PMIOPort  Port=11  Side=Left
  B2 : PMIOPort  Port=12  Side=Left
  connections:
  Series_W5W6_2/RConn2 -- 1/RConn1
  Series_W5W6_2/LConn2 -- B1/RConn1
  6/RConn1 -- Series_W5W6_3/RConn1
  Series_W5W6_2/LConn1 -- A1/RConn1
  5/RConn1 -- Series_W5W6_2/RConn1
  Series_W5W6_3/LConn2 -- B2/RConn1
  Series_W5W6_3/LConn1 -- A2/RConn1
  4/RConn1 -- Series_W5W6_1/RConn1
  Series_W5W6_3/RConn2 -- 3/RConn1
  Series_W5W6_1/RConn2 -- 2/RConn1
  Series_W5W6_1/LConn1 -- A/RConn1
  Series_W5W6_1/LConn2 -- B/RConn1

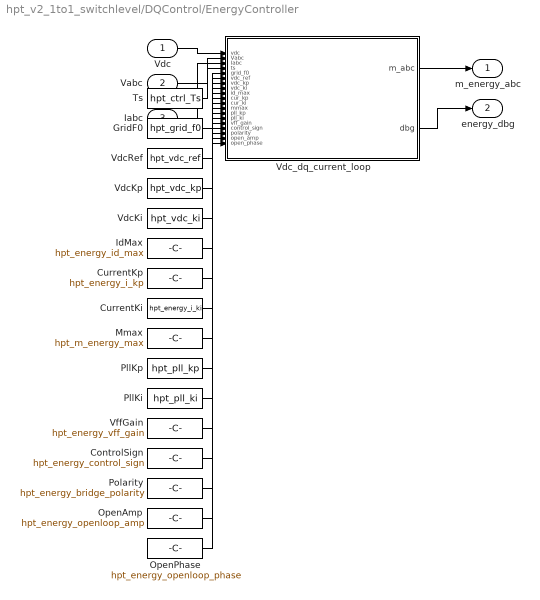
== system hpt_v2_1to1_switchlevel/DQControl/EnergyController ==
  Vdc : Inport
  Vabc : Inport  Port=2
  Iabc : Inport  Port=3
  ControlSign : Constant  Value=hpt_energy_control_sign
      mask Display: plot([20 80 80 20 20],[30 30 70 70 30]);
  CurrentKi : Constant  Value=hpt_energy_i_ki
      mask Display: plot([20 80 80 20 20],[30 30 70 70 30]);
  CurrentKp : Constant  Value=hpt_energy_i_kp
      mask Display: plot([20 80 80 20 20],[30 30 70 70 30]);
  GridF0 : Constant  Value=hpt_grid_f0
      mask Display: plot([20 80 80 20 20],[30 30 70 70 30]);
  IdMax : Constant  Value=hpt_energy_id_max
      mask Display: plot([20 80 80 20 20],[30 30 70 70 30]);
  Mmax : Constant  Value=hpt_m_energy_max
      mask Display: plot([20 80 80 20 20],[30 30 70 70 30]);
  OpenAmp : Constant  Value=hpt_energy_openloop_amp
      mask Display: plot([20 80 80 20 20],[30 30 70 70 30]);
  OpenPhase : Constant  Value=hpt_energy_openloop_phase
      mask Display: plot([20 80 80 20 20],[30 30 70 70 30]);
  PllKi : Constant  Value=hpt_pll_ki
      mask Display: plot([20 80 80 20 20],[30 30 70 70 30]);
  PllKp : Constant  Value=hpt_pll_kp
      mask Display: plot([20 80 80 20 20],[30 30 70 70 30]);
  Polarity : Constant  Value=hpt_energy_bridge_polarity
      mask Display: plot([20 80 80 20 20],[30 30 70 70 30]);
  Ts : Constant  Value=hpt_ctrl_Ts
      mask Display: plot([20 80 80 20 20],[30 30 70 70 30]);
  VdcKi : Constant  Value=hpt_vdc_ki
      mask Display: plot([20 80 80 20 20],[30 30 70 70 30]);
  VdcKp : Constant  Value=hpt_vdc_kp
      mask Display: plot([20 80 80 20 20],[30 30 70 70 30]);
  VdcRef : Constant  Value=hpt_vdc_ref
      mask Display: plot([20 80 80 20 20],[30 30 70 70 30]);
  Vdc_dq_current_loop : MATLAB Function  TreatAsAtomicUnit=on
  VffGain : Constant  Value=hpt_energy_vff_gain
      mask Display: plot([20 80 80 20 20],[30 30 70 70 30]);
  m_energy_abc : Outport
  energy_dbg : Outport  Port=2
  wires:
  Ts/1 -> Vdc_dq_current_loop/4(ts)
  GridF0/1 -> Vdc_dq_current_loop/5(grid_f0)
  VdcRef/1 -> Vdc_dq_current_loop/6(vdc_ref)
  VdcKp/1 -> Vdc_dq_current_loop/7(vdc_kp)
  VdcKi/1 -> Vdc_dq_current_loop/8(vdc_ki)
  IdMax/1 -> Vdc_dq_current_loop/9(id_max)
  CurrentKp/1 -> Vdc_dq_current_loop/10(cur_kp)
  CurrentKi/1 -> Vdc_dq_current_loop/11(cur_ki)
  Mmax/1 -> Vdc_dq_current_loop/12(mmax)
  PllKp/1 -> Vdc_dq_current_loop/13(pll_kp)
  PllKi/1 -> Vdc_dq_current_loop/14(pll_ki)
  VffGain/1 -> Vdc_dq_current_loop/15(vff_gain)
  ControlSign/1 -> Vdc_dq_current_loop/16(control_sign)
  Polarity/1 -> Vdc_dq_current_loop/17(polarity)
  OpenAmp/1 -> Vdc_dq_current_loop/18(open_amp)
  OpenPhase/1 -> Vdc_dq_current_loop/19(open_phase)
  Vdc/1 -> Vdc_dq_current_loop/1(vdc)
  Vabc/1 -> Vdc_dq_current_loop/2(Vabc)
  Iabc/1 -> Vdc_dq_current_loop/3(Iabc)
  Vdc_dq_current_loop/1(m_abc) -> m_energy_abc/1
  Vdc_dq_current_loop/2(dbg) -> energy_dbg/1

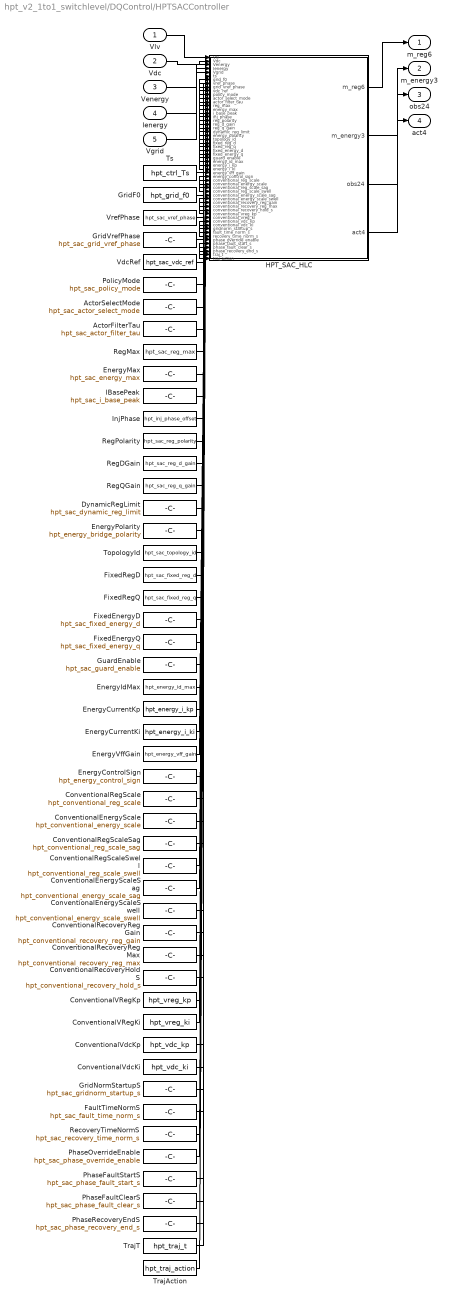
== system hpt_v2_1to1_switchlevel/DQControl/HPTSACController ==
  Vlv : Inport
  Vdc : Inport  Port=2
  Venergy : Inport  Port=3
  Ienergy : Inport  Port=4
  Vgrid : Inport  Port=5
  ActorFilterTau : Constant  Value=hpt_sac_actor_filter_tau
      mask Display: plot([20 80 80 20 20],[30 30 70 70 30]);
  ActorSelectMode : Constant  Value=hpt_sac_actor_select_mode
      mask Display: plot([20 80 80 20 20],[30 30 70 70 30]);
  ConventionalEnergyScale : Constant  Value=hpt_conventional_energy_scale
      mask Display: plot([20 80 80 20 20],[30 30 70 70 30]);
  ConventionalEnergyScaleSag : Constant  Value=hpt_conventional_energy_scale_sag
      mask Display: plot([20 80 80 20 20],[30 30 70 70 30]);
  ConventionalEnergyScaleSwell : Constant  Value=hpt_conventional_energy_scale_swell
      mask Display: plot([20 80 80 20 20],[30 30 70 70 30]);
  ConventionalRecoveryHoldS : Constant  Value=hpt_conventional_recovery_hold_s
      mask Display: plot([20 80 80 20 20],[30 30 70 70 30]);
  ConventionalRecoveryRegGain : Constant  Value=hpt_conventional_recovery_reg_gain
      mask Display: plot([20 80 80 20 20],[30 30 70 70 30]);
  ConventionalRecoveryRegMax : Constant  Value=hpt_conventional_recovery_reg_max
      mask Display: plot([20 80 80 20 20],[30 30 70 70 30]);
  ConventionalRegScale : Constant  Value=hpt_conventional_reg_scale
      mask Display: plot([20 80 80 20 20],[30 30 70 70 30]);
  ConventionalRegScaleSag : Constant  Value=hpt_conventional_reg_scale_sag
      mask Display: plot([20 80 80 20 20],[30 30 70 70 30]);
  ConventionalRegScaleSwell : Constant  Value=hpt_conventional_reg_scale_swell
      mask Display: plot([20 80 80 20 20],[30 30 70 70 30]);
  ConventionalVRegKi : Constant  Value=hpt_vreg_ki
      mask Display: plot([20 80 80 20 20],[30 30 70 70 30]);
  ConventionalVRegKp : Constant  Value=hpt_vreg_kp
      mask Display: plot([20 80 80 20 20],[30 30 70 70 30]);
  ConventionalVdcKi : Constant  Value=hpt_vdc_ki
      mask Display: plot([20 80 80 20 20],[30 30 70 70 30]);
  ConventionalVdcKp : Constant  Value=hpt_vdc_kp
      mask Display: plot([20 80 80 20 20],[30 30 70 70 30]);
  DynamicRegLimit : Constant  Value=hpt_sac_dynamic_reg_limit
      mask Display: plot([20 80 80 20 20],[30 30 70 70 30]);
  EnergyControlSign : Constant  Value=hpt_energy_control_sign
      mask Display: plot([20 80 80 20 20],[30 30 70 70 30]);
  EnergyCurrentKi : Constant  Value=hpt_energy_i_ki
      mask Display: plot([20 80 80 20 20],[30 30 70 70 30]);
  EnergyCurrentKp : Constant  Value=hpt_energy_i_kp
      mask Display: plot([20 80 80 20 20],[30 30 70 70 30]);
  EnergyIdMax : Constant  Value=hpt_energy_id_max
      mask Display: plot([20 80 80 20 20],[30 30 70 70 30]);
  EnergyMax : Constant  Value=hpt_sac_energy_max
      mask Display: plot([20 80 80 20 20],[30 30 70 70 30]);
  EnergyPolarity : Constant  Value=hpt_energy_bridge_polarity
      mask Display: plot([20 80 80 20 20],[30 30 70 70 30]);
  EnergyVffGain : Constant  Value=hpt_energy_vff_gain
      mask Display: plot([20 80 80 20 20],[30 30 70 70 30]);
  FaultTimeNormS : Constant  Value=hpt_sac_fault_time_norm_s
      mask Display: plot([20 80 80 20 20],[30 30 70 70 30]);
  FixedEnergyD : Constant  Value=hpt_sac_fixed_energy_d
      mask Display: plot([20 80 80 20 20],[30 30 70 70 30]);
  FixedEnergyQ : Constant  Value=hpt_sac_fixed_energy_q
      mask Display: plot([20 80 80 20 20],[30 30 70 70 30]);
  FixedRegD : Constant  Value=hpt_sac_fixed_reg_d
      mask Display: plot([20 80 80 20 20],[30 30 70 70 30]);
  FixedRegQ : Constant  Value=hpt_sac_fixed_reg_q
      mask Display: plot([20 80 80 20 20],[30 30 70 70 30]);
  GridF0 : Constant  Value=hpt_grid_f0
      mask Display: plot([20 80 80 20 20],[30 30 70 70 30]);
  GridNormStartupS : Constant  Value=hpt_sac_gridnorm_startup_s
      mask Display: plot([20 80 80 20 20],[30 30 70 70 30]);
  GridVrefPhase : Constant  Value=hpt_sac_grid_vref_phase
      mask Display: plot([20 80 80 20 20],[30 30 70 70 30]);
  GuardEnable : Constant  Value=hpt_sac_guard_enable
      mask Display: plot([20 80 80 20 20],[30 30 70 70 30]);
  HPT_SAC_HLC : MATLAB Function  TreatAsAtomicUnit=on
  IBasePeak : Constant  Value=hpt_sac_i_base_peak
      mask Display: plot([20 80 80 20 20],[30 30 70 70 30]);
  InjPhase : Constant  Value=hpt_inj_phase_offset
      mask Display: plot([20 80 80 20 20],[30 30 70 70 30]);
  PhaseFaultClearS : Constant  Value=hpt_sac_phase_fault_clear_s
      mask Display: plot([20 80 80 20 20],[30 30 70 70 30]);
  PhaseFaultStartS : Constant  Value=hpt_sac_phase_fault_start_s
      mask Display: plot([20 80 80 20 20],[30 30 70 70 30]);
  PhaseOverrideEnable : Constant  Value=hpt_sac_phase_override_enable
      mask Display: plot([20 80 80 20 20],[30 30 70 70 30]);
  PhaseRecoveryEndS : Constant  Value=hpt_sac_phase_recovery_end_s
      mask Display: plot([20 80 80 20 20],[30 30 70 70 30]);
  PolicyMode : Constant  Value=hpt_sac_policy_mode
      mask Display: plot([20 80 80 20 20],[30 30 70 70 30]);
  RecoveryTimeNormS : Constant  Value=hpt_sac_recovery_time_norm_s
      mask Display: plot([20 80 80 20 20],[30 30 70 70 30]);
  RegDGain : Constant  Value=hpt_sac_reg_d_gain
      mask Display: plot([20 80 80 20 20],[30 30 70 70 30]);
  RegMax : Constant  Value=hpt_sac_reg_max
      mask Display: plot([20 80 80 20 20],[30 30 70 70 30]);
  RegPolarity : Constant  Value=hpt_sac_reg_polarity
      mask Display: plot([20 80 80 20 20],[30 30 70 70 30]);
  RegQGain : Constant  Value=hpt_sac_reg_q_gain
      mask Display: plot([20 80 80 20 20],[30 30 70 70 30]);
  TopologyId : Constant  Value=hpt_sac_topology_id
      mask Display: plot([20 80 80 20 20],[30 30 70 70 30]);
  TrajAction : Constant  Value=hpt_traj_action
      mask Display: plot([20 80 80 20 20],[30 30 70 70 30]);
  TrajT : Constant  Value=hpt_traj_t
      mask Display: plot([20 80 80 20 20],[30 30 70 70 30]);
  Ts : Constant  Value=hpt_ctrl_Ts
      mask Display: plot([20 80 80 20 20],[30 30 70 70 30]);
  VdcRef : Constant  Value=hpt_sac_vdc_ref
      mask Display: plot([20 80 80 20 20],[30 30 70 70 30]);
  VrefPhase : Constant  Value=hpt_sac_vref_phase
      mask Display: plot([20 80 80 20 20],[30 30 70 70 30]);
  m_reg6 : Outport
  m_energy3 : Outport  Port=2
  obs24 : Outport  Port=3
  act4 : Outport  Port=4
  wires:
  Ts/1 -> HPT_SAC_HLC/6(ts)
  GridF0/1 -> HPT_SAC_HLC/7(grid_f0)
  VrefPhase/1 -> HPT_SAC_HLC/8(vref_phase)
  GridVrefPhase/1 -> HPT_SAC_HLC/9(grid_vref_phase)
  VdcRef/1 -> HPT_SAC_HLC/10(vdc_ref)
  PolicyMode/1 -> HPT_SAC_HLC/11(policy_mode)
  ActorSelectMode/1 -> HPT_SAC_HLC/12(actor_select_mode)
  ActorFilterTau/1 -> HPT_SAC_HLC/13(actor_filter_tau)
  RegMax/1 -> HPT_SAC_HLC/14(reg_max)
  EnergyMax/1 -> HPT_SAC_HLC/15(energy_max)
  IBasePeak/1 -> HPT_SAC_HLC/16(i_base_peak)
  InjPhase/1 -> HPT_SAC_HLC/17(inj_phase)
  RegPolarity/1 -> HPT_SAC_HLC/18(reg_polarity)
  RegDGain/1 -> HPT_SAC_HLC/19(reg_d_gain)
  RegQGain/1 -> HPT_SAC_HLC/20(reg_q_gain)
  DynamicRegLimit/1 -> HPT_SAC_HLC/21(dynamic_reg_limit)
  EnergyPolarity/1 -> HPT_SAC_HLC/22(energy_polarity)
  TopologyId/1 -> HPT_SAC_HLC/23(topology_id)
  FixedRegD/1 -> HPT_SAC_HLC/24(fixed_reg_d)
  FixedRegQ/1 -> HPT_SAC_HLC/25(fixed_reg_q)
  FixedEnergyD/1 -> HPT_SAC_HLC/26(fixed_energy_d)
  FixedEnergyQ/1 -> HPT_SAC_HLC/27(fixed_energy_q)
  GuardEnable/1 -> HPT_SAC_HLC/28(guard_enable)
  EnergyIdMax/1 -> HPT_SAC_HLC/29(energy_id_max)
  EnergyCurrentKp/1 -> HPT_SAC_HLC/30(energy_i_kp)
  EnergyCurrentKi/1 -> HPT_SAC_HLC/31(energy_i_ki)
  EnergyVffGain/1 -> HPT_SAC_HLC/32(energy_vff_gain)
  EnergyControlSign/1 -> HPT_SAC_HLC/33(energy_control_sign)
  ConventionalRegScale/1 -> HPT_SAC_HLC/34(conventional_reg_scale)
  ConventionalEnergyScale/1 -> HPT_SAC_HLC/35(conventional_energy_scale)
  ConventionalRegScaleSag/1 -> HPT_SAC_HLC/36(conventional_reg_scale_sag)
  ConventionalRegScaleSwell/1 -> HPT_SAC_HLC/37(conventional_reg_scale_swell)
  ConventionalEnergyScaleSag/1 -> HPT_SAC_HLC/38(conventional_energy_scale_sag)
  ConventionalEnergyScaleSwell/1 -> HPT_SAC_HLC/39(conventional_energy_scale_swell)
  ConventionalRecoveryRegGain/1 -> HPT_SAC_HLC/40(conventional_recovery_reg_gain)
  ConventionalRecoveryRegMax/1 -> HPT_SAC_HLC/41(conventional_recovery_reg_max)
  ConventionalRecoveryHoldS/1 -> HPT_SAC_HLC/42(conventional_recovery_hold_s)
  ConventionalVRegKp/1 -> HPT_SAC_HLC/43(conventional_vreg_kp)
  ConventionalVRegKi/1 -> HPT_SAC_HLC/44(conventional_vreg_ki)
  ConventionalVdcKp/1 -> HPT_SAC_HLC/45(conventional_vdc_kp)
  ConventionalVdcKi/1 -> HPT_SAC_HLC/46(conventional_vdc_ki)
  GridNormStartupS/1 -> HPT_SAC_HLC/47(gridnorm_startup_s)
  FaultTimeNormS/1 -> HPT_SAC_HLC/48(fault_time_norm_s)
  RecoveryTimeNormS/1 -> HPT_SAC_HLC/49(recovery_time_norm_s)
  PhaseOverrideEnable/1 -> HPT_SAC_HLC/50(phase_override_enable)
  PhaseFaultStartS/1 -> HPT_SAC_HLC/51(phase_fault_start_s)
  PhaseFaultClearS/1 -> HPT_SAC_HLC/52(phase_fault_clear_s)
  PhaseRecoveryEndS/1 -> HPT_SAC_HLC/53(phase_recovery_end_s)
  TrajT/1 -> HPT_SAC_HLC/54(traj_t)
  TrajAction/1 -> HPT_SAC_HLC/55(traj_action)
  Vlv/1 -> HPT_SAC_HLC/1(Vlv)
  Vdc/1 -> HPT_SAC_HLC/2(Vdc)
  Venergy/1 -> HPT_SAC_HLC/3(Venergy)
  Ienergy/1 -> HPT_SAC_HLC/4(Ienergy)
  Vgrid/1 -> HPT_SAC_HLC/5(Vgrid)
  HPT_SAC_HLC/1(m_reg6) -> m_reg6/1
  HPT_SAC_HLC/2(m_energy3) -> m_energy3/1
  HPT_SAC_HLC/3(obs24) -> obs24/1
  HPT_SAC_HLC/4(act4) -> act4/1

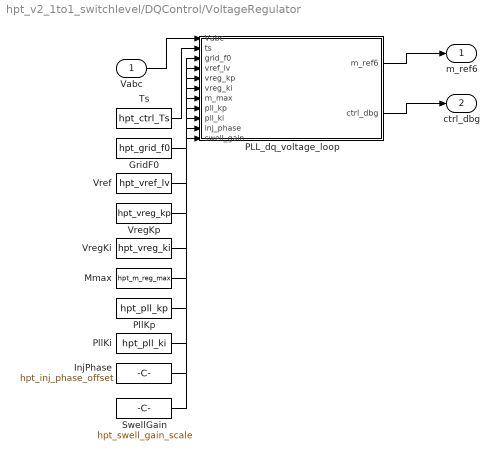
== system hpt_v2_1to1_switchlevel/DQControl/VoltageRegulator ==
  Vabc : Inport
  GridF0 : Constant  Value=hpt_grid_f0
      mask Display: plot([20 80 80 20 20],[30 30 70 70 30]);
  InjPhase : Constant  Value=hpt_inj_phase_offset
      mask Display: plot([20 80 80 20 20],[30 30 70 70 30]);
  Mmax : Constant  Value=hpt_m_reg_max
      mask Display: plot([20 80 80 20 20],[30 30 70 70 30]);
  PLL_dq_voltage_loop : MATLAB Function  TreatAsAtomicUnit=on
  PllKi : Constant  Value=hpt_pll_ki
      mask Display: plot([20 80 80 20 20],[30 30 70 70 30]);
  PllKp : Constant  Value=hpt_pll_kp
      mask Display: plot([20 80 80 20 20],[30 30 70 70 30]);
  SwellGain : Constant  Value=hpt_swell_gain_scale
      mask Display: plot([20 80 80 20 20],[30 30 70 70 30]);
  Ts : Constant  Value=hpt_ctrl_Ts
      mask Display: plot([20 80 80 20 20],[30 30 70 70 30]);
  Vref : Constant  Value=hpt_vref_lv
      mask Display: plot([20 80 80 20 20],[30 30 70 70 30]);
  VregKi : Constant  Value=hpt_vreg_ki
      mask Display: plot([20 80 80 20 20],[30 30 70 70 30]);
  VregKp : Constant  Value=hpt_vreg_kp
      mask Display: plot([20 80 80 20 20],[30 30 70 70 30]);
  m_ref6 : Outport
  ctrl_dbg : Outport  Port=2
  wires:
  Ts/1 -> PLL_dq_voltage_loop/2(ts)
  GridF0/1 -> PLL_dq_voltage_loop/3(grid_f0)
  Vref/1 -> PLL_dq_voltage_loop/4(vref_lv)
  VregKp/1 -> PLL_dq_voltage_loop/5(vreg_kp)
  VregKi/1 -> PLL_dq_voltage_loop/6(vreg_ki)
  Mmax/1 -> PLL_dq_voltage_loop/7(m_max)
  PllKp/1 -> PLL_dq_voltage_loop/8(pll_kp)
  PllKi/1 -> PLL_dq_voltage_loop/9(pll_ki)
  InjPhase/1 -> PLL_dq_voltage_loop/10(inj_phase)
  SwellGain/1 -> PLL_dq_voltage_loop/11(swell_gain)
  Vabc/1 -> PLL_dq_voltage_loop/1(Vabc)
  PLL_dq_voltage_loop/1(m_ref6) -> m_ref6/1
  PLL_dq_voltage_loop/2(ctrl_dbg) -> ctrl_dbg/1
